simulink model "ad_blackbox"  (R2015b)
settings: Solver=FixedStepDiscrete  SolverMode=SingleTasking  StartTime=0.0  StopTime=1  RelTol=1e-3
libraries: simulink x2, dspxfrm3 x1
settings Model: Creator=at-mt  LastModifiedBy=amatsumo
settings DataIOCC: SaveFormat=Array  SignalLoggingSaveFormat=ModelDataLogs  SaveOutput=off  SignalLogging=off  SaveTime=off
settings OptimizationCC: BlockReduction=off  ConditionallyExecuteInputs=off  DefaultParameterBehavior=Inlined  ExpressionDepthLimit=2147483647
settings DebuggingCC: AlgebraicLoopMsg=error  UnderspecifiedInitializationDetection=Classic  MergeDetectMultiDrivingBlocksExec=none  SolverPrmCheckMsg=warning  SingleTaskRateTransMsg=error  FcnCallInpInsideContextMsg=UseLocalSettings  StateNameClashWarn=warning
settings HardwareCC: ProdBitPerPointer=32  ProdLargestAtomicFloat=None  ProdIntDivRoundTo=Undefined  ProdEndianess=Unspecified  ProdWordSize=32  ProdHWDeviceType=ASIC/FPGA->ASIC/FPGA  ProdEqTarget=off
settings SFSimCC: SFSimEcho=off
settings GRTTargetCC: GeneratePreprocessorConditionals=Disable all  CombineOutputUpdateFcns=off  GRTInterface=on
settings ConfigComp: CovModelRefEnable=Off  CovSFcnEnable=off

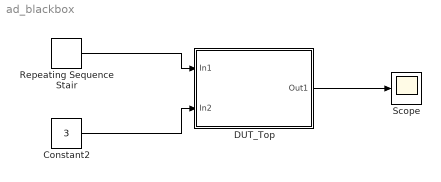
== system ad_blackbox ==
  Constant2 : Constant  Value=3  OutDataTypeStr=int8  SampleTime=0.01
  DUT_Top : Subsystem
  Repeating Sequence Stair : simulink/Sources/Repeating Sequence Stair  OutValues=[3 1 4 2 1].'  tsamp=0.01  OutMin=[]  OutMax=[]  OutDataTypeStr=int8  OutputDataTypeScalingMode=int8  OutDataType=double  ConRadixGroup=Best Precision: Vector-wise  OutScaling=2^-12
  Scope : Scope
  wires:
  Repeating Sequence Stair/1 -> DUT_Top/1(In1)
  Constant2/1 -> DUT_Top/2(In2)
  DUT_Top/1(Out1) -> Scope/1

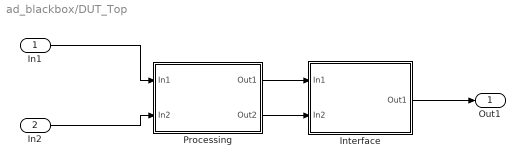
== system ad_blackbox/DUT_Top ==
  In1 : Inport
  In2 : Inport  Port=2
  Interface : Subsystem
  Processing : Subsystem
  Out1 : Outport
  wires:
  Processing/1(Out1) -> Interface/1(In1)
  In1/1 -> Processing/1(In1)
  Interface/1(Out1) -> Out1/1
  In2/1 -> Processing/2(In2)
  Processing/2(Out2) -> Interface/2(In2)

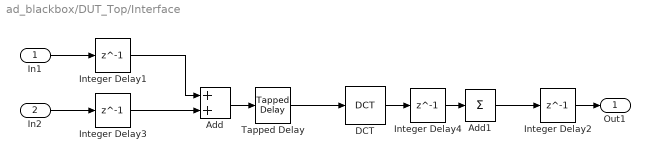
== system ad_blackbox/DUT_Top/Interface ==
  In1 : Inport
  In2 : Inport  Port=2
  Add : Sum
  Add1 : Sum  Inputs=+
  DCT : dspxfrm3/DCT  CompMethod=Table lookup  roundingMode=Floor  overflowMode=off  firstCoeffDataTypeStr=Inherit: Same word length as input  firstCoeffLastDataTypeStr=Inherit: Same word length as input  outputMin=[]  outputMax=[]
  Integer Delay{1..4} (4 alike) : Delay  DelayLength=1  InputProcessing=Inherited
  Tapped Delay : simulink/Discrete/Tapped Delay  vinit=0.0  samptime=-1  NumDelays=31  DelayOrder=Newest  includeCurrent=on
  Out1 : Outport
  wires:
  DCT/1 -> Integer Delay4/1
  In1/1 -> Integer Delay1/1
  Integer Delay2/1 -> Out1/1
  In2/1 -> Integer Delay3/1
  Integer Delay1/1 -> Add/1
  Integer Delay3/1 -> Add/2
  Add/1 -> Tapped Delay/1
  Tapped Delay/1 -> DCT/1
  Add1/1 -> Integer Delay2/1
  Integer Delay4/1 -> Add1/1

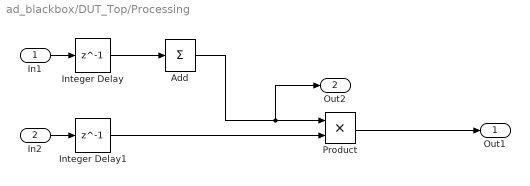
== system ad_blackbox/DUT_Top/Processing ==
  In1 : Inport
  In2 : Inport  Port=2
  Add : Sum  Inputs=+
  Integer Delay : Delay  DelayLength=1  InputProcessing=Inherited
  Integer Delay1 : Delay  DelayLength=1  InputProcessing=Inherited
  Product : Product  RndMeth=Zero
  Out1 : Outport
  Out2 : Outport  Port=2
  wires:
  Integer Delay/1 -> Add/1
  Add/1 -> Product/1, Out2/1
  Integer Delay1/1 -> Product/2
  In1/1 -> Integer Delay/1
  Product/1 -> Out1/1
  In2/1 -> Integer Delay1/1
